simulink model "mcb_stm32_param_est_host_read"  (R2024a)
settings: Solver=FixedStepDiscrete  StartTime=0.0  StopTime=60  RelTol=1e-3
InitFcn:
  | mcb_stm32_param_est_InitFunc(bdroot);
StopFcn:
  | mcb_param_est_StopFunc(bdroot);
values from neighbouring files (symbols this model uses):
  motorParam =     [matlab.mat]
  Speed_per_unit_scaler = motorParam.ratedSpeed    [mcb_stm32_param_est_InitFunc.m]
  Ts = 1/PWM_frequency    (= 5e-05)    [mcb_stm32_param_est_InitFunc.m]    (also in stm32_pmsm_foc_data.m)
undefined symbols (not defined in the file or in its folder): inverter
libraries: instrumentseriallib x5, simulink x5
settings Model: Creator=The MathWorks, Inc.  LastModifiedBy=wsl
settings SolverCC: AlgebraicLoopSolver=TrustRegion  MaxZcPerStep=1
settings DataIOCC: LimitDataPoints=on  SaveFormat=Array  ReturnWorkspaceOutputs=off
settings OptimizationCC: ReuseModelBlockBuffer=off  LifeSpan=1  EfficientTunableParamExpr=on
settings DebuggingCC: UnderspecifiedInitializationDetection=Classic  MergeDetectMultiDrivingBlocksExec=none  SolverPrmCheckMsg=warning  MultiTaskCondExecSysMsg=warning  ParameterOverflowMsg=none  ParameterPrecisionLossMsg=none  UnconnectedInputMsg=warning  UnconnectedOutputMsg=warning  UnconnectedLineMsg=warning  AllowSymbolicDim=off  SubsystemReferenceDiagnosticForUnitTest=warning  SFUnexpectedBacktrackingDiag=warning  SFNoUnconditionalDefaultTransitionDiag=warning  SFExecutionAtInitializationDiag=none  ArithmeticOperatorsInVariantConditions=warning
settings HardwareCC: ProdBitPerPointer=32  ProdLargestAtomicFloat=None  ProdIntDivRoundTo=Undefined  ProdEndianess=Unspecified  ProdWordSize=32  ProdHWDeviceType=32-bit Generic
settings ModelReferenceCC: EnableRefExpFcnMdlSchedulingChecks=on  PropagateSignalLabelsOutOfModel=off
settings SFSimCC: SimUseLocalCustomCode=off  MATLABDynamicMemAlloc=off
settings RTWCC: Description=Real-Time Workshop Embedded Coder  SystemTargetFile=ert.tlc  TemplateMakefile=ert_default_tmf  GenerateReport=on  RTWUseLocalCustomCode=off  IncludeHyperlinkInReport=on  LaunchReport=on  GenerateTraceInfo=on  GenerateTraceReport=on  GenerateTraceReportSl=on  GenerateTraceReportSf=on  GenerateTraceReportEml=on  GPUComputeCapability=3.5  DLArmComputeVersion=19.05
settings CodeAppCC: IgnoreCustomStorageClasses=off  StateflowObjectComments=on  InternalIdentifier=Classic
settings ERTTargetCC: MultiwordLength=2048  GenerateSampleERTMain=on  ERTCustomFileTemplate=example_file_process.tlc  ConvertIfToSwitch=off  SuppressUnreachableDefaultCases=off
settings ConfigComp: CovMetricSettings=dw  CovSaveCumulativeToWorkspaceVar=on  CovSaveSingleToWorkspaceVar=on  CovExternalEMLEnable=off  CovSFcnEnable=off

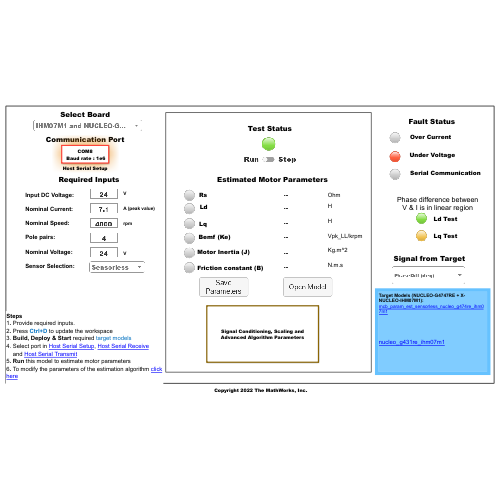
[thumbnail: Simulink's stored preview of the top-level diagram]
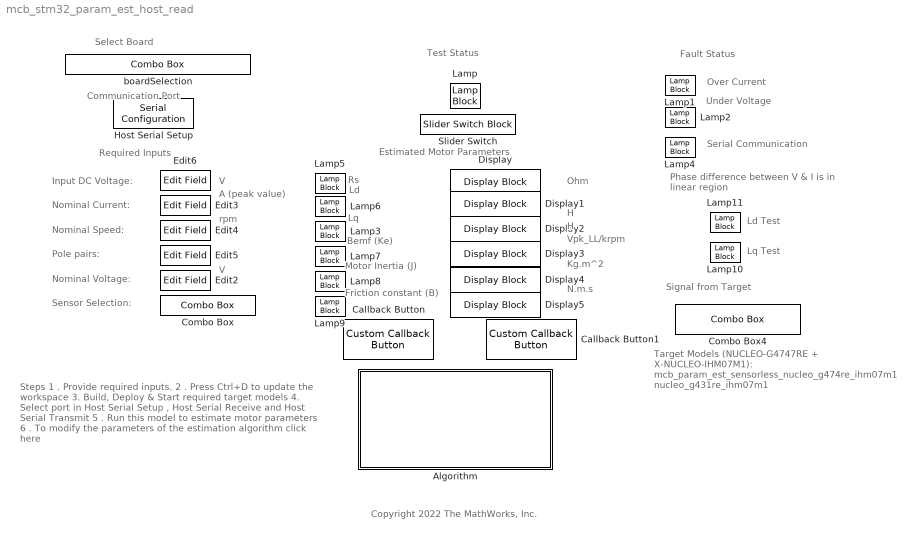
== system mcb_stm32_param_est_host_read ==
  note: Rs
  note: Ld
  note: Lq
  note: Bemf (Ke)
  note: Motor Inertia (J)
  note: Required Inputs
  note: Select Board
  note: Nominal Voltage:
  note: Nominal Current:
  note: Nominal Speed:
  note: rpm
  note: V
  note: A (peak value)
  note: Pole pairs:
  note: Input DC Voltage:
  note: Friction constant (B)
  note: Ohm
  note: H
  note: N.m.s
  note: Over Current
  note: Under Voltage
  note: Serial Communication
  note: Estimated Motor Parameters
  note: Signal from Target
  note: Test Status
  note: Copyright 2022 The MathWorks, Inc.
  note: Communication Port
  note: Sensor Selection:
  note: Steps
      | 1 . Provide required inputs.
      | 2 . Press Ctrl+D to update the workspace
      | 3. Build, Deploy & Start required target models
      | 4. Select port in Host Serial Setup , Host Serial Receive
      | and Host Serial Transmit
      | 5 . Run this model to estimate motor parameters
      | 6 . To modify the parameters of the estimation algorithm click here
  note: Vpk_LL/krpm
  note: H
  note: Kg.m^2
  note: V
  note: Target Models (NUCLEO-G4747RE + X-NUCLEO-IHM07M1):
      | mcb_param_est_sensorless_nucleo_g474re_ihm07m1
      |
      | nucleo_g431re_ihm07m1
  note: Phase difference between
      | V & I is in linear region
  note: Ld Test
  note: Lq Test
  note: Fault Status
  Algorithm : Subsystem
      mask Display: fprintf('Signal Conditioning, Scaling and\nAdvanced Algorithm Parameters')
  Callback Button : CustomCallbackButton  Configuration="{\"components\":[{\"name\":\"BackgroundImageComponent\",\"settings\":{\"image\":{\"size\":[0,0],\"src\":\"default\",\"srcOrientation\":\"Right\"},\"position\":[0,0,1,1]}},{\"name\":\"ButtonStateComponent\",\"settings\":{\"buttonType\":\"momentary\",\"clickFcn\":\"uisave('motorParam');\",\"onValue\":1,\"position\":[0,0,1,1],\"pressDelay\":\"500\",\"pressFcn\":\"\",\"repeatInterval\":\"0\",\"states\":[{\"horizontalAlignment\":\"center\",\"image\":{\"position\":[0,0,1,1],\"src\":\"default\",\"srcOrientation\":\"Right\"},\"label\":{\"color\":[0.01176470588,0.01176470588,0.01176470588,1],\"icon\":{\"size\":[0,0],\"src\":\"default\",\"srcOrientation\":\"Right\"},\"iconPlacement\":\"left\",\"text\":{\"content\":\"Save Parameters\"}},\"labelOffset\":[0,0],\"verticalAlignment\":\"middle\"},{\"horizontalAlignment\":\"center\",\"image\":{\"position\":[0,0,1,1],\"src\":\"default\",\"srcOrientation\":\"Right\"},\"label\":{\"color\":[0.01176470588,0.01176470588,0.01176470588,1],\"icon\":{\"size\":[0,0],\"src\":\"default\",\"srcOrientation\":\"Right\"},\"iconPlacement\":\"left\",\"text\":{\"content\":\"Save Parameters\"}},\"labelOffset\":[0,0],\"verticalAlignment\":\"middle\"},{\"horizontalAlignment\":\"center\",\"image\":{\"position\":[0,0,1,1],\"src\":\"default\",\"srcOrientation\":\"Right\"},\"label\":{\"color\":[0.01176470588,0.01176470588,0.01176470588,1],\"icon\":{\"size\":[0,0],\"src\":\"default\",\"srcOrientation\":\"Right\"},\"iconPlacement\":\"left\",\"text\":{\"content\":\"Save Parameters\"}},\"labelOffset\":[0,0],\"verticalAlignment\":\"middle\"},{\"horizontalAlignment\":\"center\",\"image\":{\"position\":[0,0,1,1],\"src\":\"default\",\"srcOrientation\":\"Right\"},\"label\":{\"color\":[0.01176470588,0.01176470588,0.01176470588,1],\"icon\":{\"size\":[0,0],\"src\":\"default\",\"srcOrientation\":\"Right\"},\"iconPlacement\":\"left\",\"text\":{\"content\":\"Save Parameters\"}},\"labelOffset\":[0,0],\"verticalAlignment\":\"middle\"}]}},{\"name\":\"ForegroundImageComponent\",\"settings\":{\"image\":{\"size\":[0,0],\"src\":\"default\",\"srcOrientation\":\"Right\"},\"isForeground\":1,\"position\":[0,0,1,1]}}],\"settings\":{\"BindingType\":\"standalone\",\"backgroundColor\":[244,244,244,1],\"backgroundOffset\":0.2,\"backgroundOpacity\":1,\"fixedAspectRatio\":\"off\",\"foregroundColor\":[0.01176470588,0.01176470588,0.01176470588,1],\"migratedFromLegacy\":true,\"useBackgroundColor\":true,\"variant\":\"callback\",\"version\":\"R2023a\"},\"type\":\"Button\"}"  CustomBackgroundColor="{\"color\":[0.9568627451,0.9568627451,0.9568627451],\"show\":true}"
  Callback Button1 : CustomCallbackButton  Configuration="{\"components\":[{\"name\":\"BackgroundImageComponent\",\"settings\":{\"image\":{\"size\":[0,0],\"src\":\"default\",\"srcOrientation\":\"Right\"},\"position\":[0,0,1,1]}},{\"name\":\"ButtonStateComponent\",\"settings\":{\"buttonType\":\"momentary\",\"clickFcn\":\"hdl = new_system;\\nopen_system(hdl);\\nblkHdl = add_block('mcblib\\/Electrical Systems\\/Motors\\/Interior PMSM', [get_param(hdl,'Name'),'\\/Interior PMSM']);\\nopen_system(hdl);\\nset_param(blkHdl,'P','motorParam.p');\\nset_param(blkHdl,'Rs','motorParam.Rs');\\nset_param(blkHdl,'Ldq','[motorParam.Ld motorParam.Lq]');\\nset_param(blkHdl,'KConstText','Back-emf constant (Ke):');\\nset_param(blkHdl,'Ke','motorParam.Ke');\\nset_param(blkHdl,'mechanical','[motorParam.J, motorParam.B, 0]');\",\"onValue\":1,\"position\":[0,0,1,1],\"pressDelay\":\"500\",\"pressFcn\":\"\",\"repeatInterval\":\"0\",\"states\":[{\"horizontalAlignment\":\"center\",\"image\":{\"position\":[0,0,1,1],\"src\":\"default\",\"srcOrientation\":\"Right\"},\"label\":{\"color\":[0.01176470588,0.01176470588,0.01176470588,1],\"icon\":{\"size\":[0,0],\"src\":\"default\",\"srcOrientation\":\"Right\"},\"iconPlacement\":\"left\",\"text\":{\"content\":\"Open Model\"}},\"labelOffset\":[0,0],\"verticalAlignment\":\"middle\"},{\"horizontalAlignment\":\"center\",\"image\":{\"position\":[0,0,1,1],\"src\":\"default\",\"srcOrientation\":\"Right\"},\"label\":{\"color\":[0.01176470588,0.01176470588,0.01176470588,1],\"icon\":{\"size\":[0,0],\"src\":\"default\",\"srcOrientation\":\"Right\"},\"iconPlacement\":\"left\",\"text\":{\"content\":\"Open Model\"}},\"labelOffset\":[0,0],\"verticalAlignment\":\"middle\"},{\"horizontalAlignment\":\"center\",\"image\":{\"position\":[0,0,1,1],\"src\":\"default\",\"srcOrientation\":\"Right\"},\"label\":{\"color\":[0.01176470588,0.01176470588,0.01176470588,1],\"icon\":{\"size\":[0,0],\"src\":\"default\",\"srcOrientation\":\"Right\"},\"iconPlacement\":\"left\",\"text\":{\"content\":\"Open Model\"}},\"labelOffset\":[0,0],\"verticalAlignment\":\"middle\"},{\"horizontalAlignment\":\"center\",\"image\":{\"position\":[0,0,1,1],\"src\":\"default\",\"srcOrientation\":\"Right\"},\"label\":{\"color\":[0.01176470588,0.01176470588,0.01176470588,1],\"icon\":{\"size\":[0,0],\"src\":\"default\",\"srcOrientation\":\"Right\"},\"iconPlacement\":\"left\",\"text\":{\"content\":\"Open Model\"}},\"labelOffset\":[0,0],\"verticalAlignment\":\"middle\"}]}},{\"name\":\"ForegroundImageComponent\",\"settings\":{\"image\":{\"size\":[0,0],\"src\":\"default\",\"srcOrientation\":\"Right\"},\"isForeground\":1,\"position\":[0,0,1,1]}}],\"settings\":{\"BindingType\":\"standalone\",\"backgroundColor\":[244,244,244,1],\"backgroundOffset\":0.2,\"backgroundOpacity\":1,\"fixedAspectRatio\":\"off\",\"foregroundColor\":[0.01176470588,0.01176470588,0.01176470588,1],\"migratedFromLegacy\":true,\"useBackgroundColor\":true,\"variant\":\"callback\",\"version\":\"R2023a\"},\"type\":\"Button\"}"  CustomBackgroundColor="{\"color\":[0.9568627451,0.9568627451,0.9568627451],\"show\":true}"
  Combo Box : ComboBox  LabelPosition=Hide  SelectedLabel=Sensorless
      settings: Values={{'Sensorless'}, 2}
  Combo Box4 : ComboBox  LabelPosition=Hide  SelectedLabel=PhaseDiff (deg)
      settings: Values={{'Vd', 'Id', 'Vq', 'Iq', 'Ia', 'Ib', 'Theta', 'Speed', 'Vq_Meas', 'Vd_Meas', 'Vdc_Meas', 'PhaseDiff (deg)'}, [1 8 0 7 9 10 6 5 3 4 2 11]}
  Display{,1..5} (6 alike) : DisplayBlock  LabelPosition=Hide  Transparency=1  Opacity=0.001
  Edit{2..6} (5 alike) : EditField  LabelPosition=Hide  ShowInitialText=on  Alignment=Center
  Host Serial Setup : instrumentseriallib/Serial Configuration  Priority=-99  PortSel=COM8  Port=COM8  ComPort=COM8  BaudRate=1e6  DataBits=8  Parity=none  StopBits=1  ByteOrder=little-endian  FlowControl=none  Timeout=1  SimulateUsing=Interpreted execution  BlockInModel=on  aMode=5
  Lamp{,1..11} (12 alike) : LampBlock  LabelPosition=Hide
  Slider Switch : SliderSwitchBlock  LabelPosition=Hide
      settings: Values={{'Run', 'Stop'}, [1 0]}
  boardSelection : ComboBox  LabelPosition=Hide  SelectedLabel=IHM07M1 and NUCLEO-G474RE
      settings: Values={{'IHM07M1 and NUCLEO-G474RE'}, 2}

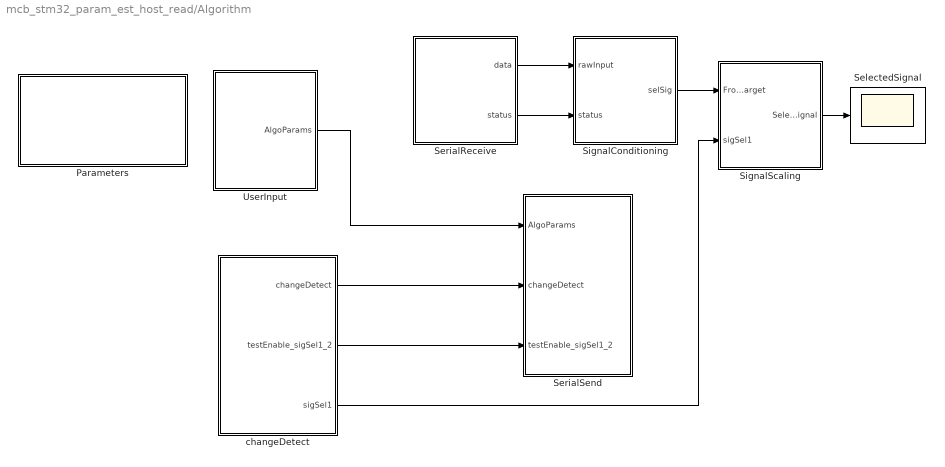
== system mcb_stm32_param_est_host_read/Algorithm ==
  Parameters : Subsystem
      mask Display: fprintf('Advanced Algorithm Parameters')
  SelectedSignal : Scope
  SerialReceive : Subsystem  Variant=on  VariantControlMode=label  LabelModeActiveChoice=Floating_Point_Target
  SerialSend : Subsystem  VariantControl=Choice
  SignalConditioning : Subsystem
  SignalScaling : Subsystem
  UserInput : Subsystem
  changeDetect : Subsystem
  wires:
  changeDetect/1(changeDetect) -> SerialSend/2(changeDetect)
  changeDetect/2("testEnable_sigSel1_2 ") -> SerialSend/3(testEnable_sigSel1_2)
  changeDetect/3(sigSel1) -> SignalScaling/2(sigSel1)
  SignalConditioning/1(selSig) -> SignalScaling/1(FromTarget)
  UserInput/1(AlgoParams) -> SerialSend/1(AlgoParams)
  SerialReceive/1(data) -> SignalConditioning/1(rawInput)
  SerialReceive/2(status) -> SignalConditioning/2(status)
  SignalScaling/1(SelectedSignal) -> SelectedSignal/1

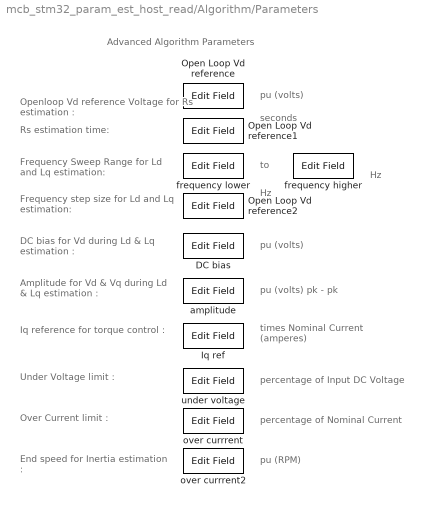
== system mcb_stm32_param_est_host_read/Algorithm/Parameters ==
  note: Openloop Vd reference Voltage
      | for Rs estimation :
  note: pu (volts)
  note: Frequency Sweep Range for Ld and Lq estimation:
  note: to
  note: Hz
  note: DC bias for Vd during Ld & Lq estimation :
  note: Amplitude for Vd & Vq during Ld & Lq estimation :
  note: Iq reference for torque control :
  note: times Nominal Current (amperes)
  note: Under Voltage limit :
  note: percentage of Input DC Voltage
  note: Over Current limit :
  note: percentage of Nominal Current
  note: Rs estimation time:
  note: seconds
  note: Advanced Algorithm Parameters
  note: Frequency step size for Ld and Lq estimation:
  note: Hz
  note: End speed for Inertia estimation :
  note: pu (RPM)
  note: pu (volts)
  note: pu (volts) pk - pk
  DC bias : EditField  LabelPosition=Hide  ShowInitialText=on  Alignment=Center
  Iq ref : EditField  LabelPosition=Hide  ShowInitialText=on  Alignment=Center
  Open Loop Vd reference : EditField  LabelPosition=Hide  ShowInitialText=on  Alignment=Center
  Open Loop Vd reference1 : EditField  LabelPosition=Hide  ShowInitialText=on  Alignment=Center
  Open Loop Vd reference2 : EditField  LabelPosition=Hide  ShowInitialText=on  Alignment=Center
  amplitude : EditField  LabelPosition=Hide  ShowInitialText=on  Alignment=Center
  frequency higher : EditField  LabelPosition=Hide  ShowInitialText=on  Alignment=Center
  frequency lower : EditField  LabelPosition=Hide  ShowInitialText=on  Alignment=Center
  over currrent : EditField  LabelPosition=Hide  ShowInitialText=on  Alignment=Center
  over currrent2 : EditField  LabelPosition=Hide  ShowInitialText=on  Alignment=Center
  under voltage : EditField  LabelPosition=Hide  ShowInitialText=on  Alignment=Center

== system mcb_stm32_param_est_host_read/Algorithm/SerialReceive ==
  Fixed_Point_Target : Subsystem  VariantControl=Fixed_Point_Target
  Floating_Point_Target : Subsystem  VariantControl=Floating_Point_Target
  data : Outport
  status : Outport  Port=2

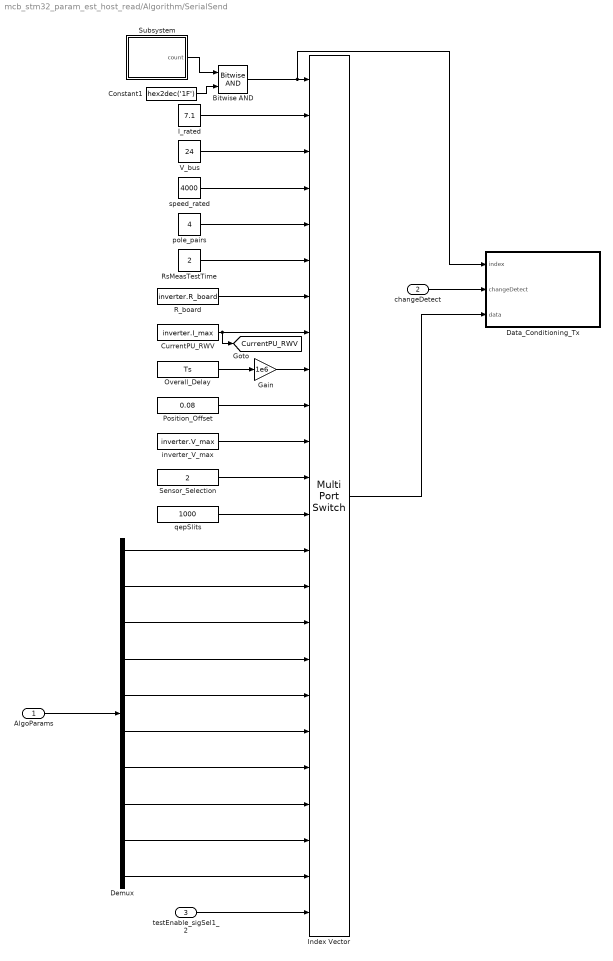
== system mcb_stm32_param_est_host_read/Algorithm/SerialSend ==
  AlgoParams : Inport
  changeDetect : Inport  Port=2
  testEnable_sigSel1_2 : Inport  Port=3
  Bitwise AND : simulink/Logic and Bit Operations/Bitwise Operator  logicop=AND  UseBitMask=off  NumInputPorts=2  BitMask=bin2dec('00001111')  BitMaskRealWorld=Stored Integer
  Constant1 : Constant  Value=hex2dec('1F')  OutDataTypeStr=uint8  SampleTime=-1
  CurrentPU_RWV : Constant  Value=inverter.I_max  OutDataTypeStr=single  SampleTime=-1
  Data_Conditioning_Tx : Subsystem  Variant=on  VariantControlMode=label  LabelModeActiveChoice=Floating_Point_Target
  Demux : Demux  Outputs=10
  Gain : Gain  Gain=1e6  OutDataTypeStr=single  RndMeth=Simplest
  I_rated : Constant  Value=7.1  OutMin=[0]  OutMax=[25000]  OutDataTypeStr=single  SampleTime=-1
  Index Vector : MultiPortSwitch  Inputs=23  OutDataTypeStr=single  RndMeth=Simplest  SaturateOnIntegerOverflow=off  InputSameDT=off
  Overall_Delay : Constant  Value=Ts  OutDataTypeStr=single  SampleTime=-1
  Position_Offset : Constant  Value=0.08  OutMin=[0]  OutMax=[1]  OutDataTypeStr=single  SampleTime=-1
  R_board : Constant  Value=inverter.R_board  OutDataTypeStr=single  SampleTime=-1
  RsMeasTestTime : Constant  Value=2  OutMin=[0.2]  OutMax=[25000]  OutDataTypeStr=single  SampleTime=-1
  Sensor_Selection : Constant  Value=2  OutDataTypeStr=single  SampleTime=-1
  Subsystem : Subsystem  mask(Counter){upperLimit=23, sampleTime=1e-3}
      mask prompts: upperLimit "Upper Limit"; sampleTime "Sample Time"
      mask help: Conter starts from 1 and reaches Upper Limit using given sample time in steps of 1.
  V_bus : Constant  Value=24  OutMin=[0]  OutMax=[25000]  OutDataTypeStr=single  SampleTime=-1
  inverter_V_max : Constant  Value=inverter.V_max  OutDataTypeStr=single  SampleTime=-1
  pole_pairs : Constant  Value=4  OutMin=[1]  OutMax=[25000]  OutDataTypeStr=single  SampleTime=-1
  qepSlits : Constant  Value=1000  OutDataTypeStr=single  SampleTime=-1
  speed_rated : Constant  Value=4000  OutMin=[0]  OutMax=[25000]  OutDataTypeStr=single  SampleTime=-1
  tag scope: CurrentPU_RWV=global
  wires:
  pole_pairs/1 -> Index Vector/5
  V_bus/1 -> Index Vector/3
  speed_rated/1 -> Index Vector/4
  Constant1/1 -> Bitwise AND/2
  RsMeasTestTime/1 -> Index Vector/6
  Bitwise AND/1 -> Data_Conditioning_Tx/1(index), Index Vector/1
  R_board/1 -> Index Vector/7
  CurrentPU_RWV/1 -> [CurrentPU_RWV], Index Vector/8
  Overall_Delay/1 -> Gain/1
  Gain/1 -> Index Vector/9
  I_rated/1 -> Index Vector/2
  inverter_V_max/1 -> Index Vector/11
  Sensor_Selection/1 -> Index Vector/12
  Position_Offset/1 -> Index Vector/10
  qepSlits/1 -> Index Vector/13
  changeDetect/1 -> Data_Conditioning_Tx/2(changeDetect)
  Index Vector/1 -> Data_Conditioning_Tx/3(data)
  AlgoParams/1 -> Demux/1
  Subsystem/1(count) -> Bitwise AND/1
  Demux/1 -> Index Vector/14
  Demux/2 -> Index Vector/15
  Demux/3 -> Index Vector/16
  Demux/4 -> Index Vector/17
  Demux/5 -> Index Vector/18
  Demux/6 -> Index Vector/19
  Demux/7 -> Index Vector/20
  Demux/8 -> Index Vector/21
  Demux/9 -> Index Vector/22
  Demux/10 -> Index Vector/23
  testEnable_sigSel1_2/1 -> Index Vector/24

== system mcb_stm32_param_est_host_read/Algorithm/SignalConditioning ==
  rawInput : Inport
  status : Inport  Port=2
  Data_Conditioning1 : MATLAB Function  TreatAsAtomicUnit=on
  Data_Conditioning2 : MATLAB Function  TreatAsAtomicUnit=on
  ErrorConditions : MATLAB Function  TreatAsAtomicUnit=on
  LatchIdx : Subsystem
  Subsystem1 : Subsystem
  selSig : Outport
  wires:
  Subsystem1/1(errorID) -> ErrorConditions/3(errorID)
  Data_Conditioning1/2(estParam) -> Subsystem1/2(estimatedParameter)
  Data_Conditioning1/1(estParamIdx) -> LatchIdx/2(estParIdx), ErrorConditions/2(idx), Subsystem1/1(Idx)
  rawInput/1 -> Data_Conditioning2/1(rawInput), Data_Conditioning1/2(rawInput)
  Data_Conditioning2/1(selSignal) -> selSig/1
  status/1 -> ErrorConditions/1(status), LatchIdx/1(status), Data_Conditioning1/1(unused)

== system mcb_stm32_param_est_host_read/Algorithm/SignalScaling ==
  FromTarget : Inport
  sigSel1 : Inport  Port=2
  Data Type Conversion : DataTypeConversion  OutDataTypeStr=single  RndMeth=Simplest  SaturateOnIntegerOverflow=off
  PU2RWV : Subsystem
  To Workspace3 : ToWorkspace  VariableName=SignalsScaled  SaveFormat=Timeseries  SampleTime=-1
  SelectedSignal : Outport
  wires:
  FromTarget/1 -> Data Type Conversion/1  "FreqTrgt/Speed"
  sigSel1/1 -> PU2RWV/2(SelTestHost)
  PU2RWV/1(RWV) -> SelectedSignal/1, To Workspace3/1  "SelectedSignal"
  Data Type Conversion/1 -> PU2RWV/1(SigFromTarget)

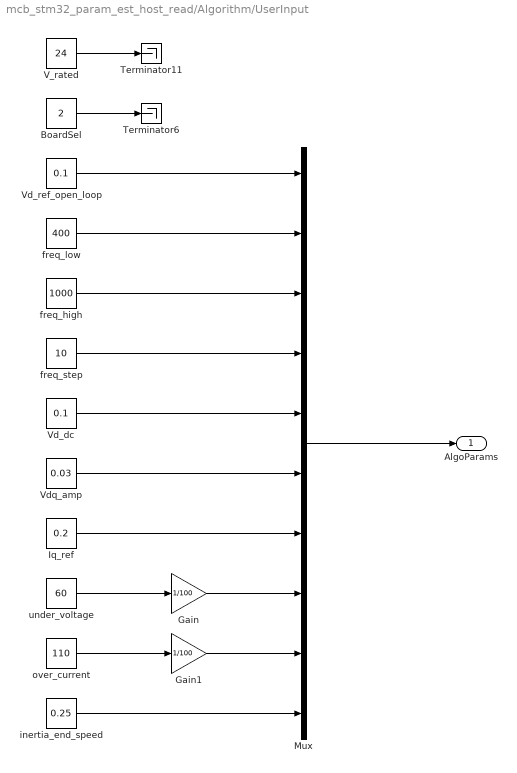
== system mcb_stm32_param_est_host_read/Algorithm/UserInput ==
  BoardSel : Constant  Value=2  OutDataTypeStr=single  SampleTime=-1
  Gain : Gain  Gain=1/100  OutDataTypeStr=single  RndMeth=Simplest
  Gain1 : Gain  Gain=1/100  OutDataTypeStr=single  RndMeth=Simplest
  Iq_ref : Constant  Value=0.2  OutMin=[0.05]  OutMax=[0.5]  OutDataTypeStr=single  SampleTime=-1
  Mux : Mux  Inputs=10
  Terminator11 : Terminator
  Terminator6 : Terminator
  V_rated : Constant  Value=24  OutMin=[0]  OutMax=[100000]  OutDataTypeStr=single  SampleTime=-1
  Vd_dc : Constant  Value=0.1  OutMin=[0.01]  OutMax=[0.5]  OutDataTypeStr=single  SampleTime=-1
  Vd_ref_open_loop : Constant  Value=0.1  OutMin=[0.01]  OutMax=[0.5]  OutDataTypeStr=single  SampleTime=-1
  Vdq_amp : Constant  Value=0.03  OutMin=[1e-3]  OutMax=[0.9]  OutDataTypeStr=single  SampleTime=-1
  freq_high : Constant  Value=1000  OutMin=[100]  OutMax=[10000]  OutDataTypeStr=single  SampleTime=-1
  freq_low : Constant  Value=400  OutMin=[100]  OutMax=[10000]  OutDataTypeStr=single  SampleTime=-1
  freq_step : Constant  Value=10  OutMin=[10]  OutMax=[10000]  OutDataTypeStr=single  SampleTime=-1
  inertia_end_speed : Constant  Value=0.25  OutMin=[0.25]  OutMax=[0.7]  OutDataTypeStr=single  SampleTime=-1
  over_current : Constant  Value=110  OutMin=[20]  OutMax=[150]  OutDataTypeStr=single  SampleTime=-1
  under_voltage : Constant  Value=60  OutMin=[10]  OutMax=[100]  OutDataTypeStr=single  SampleTime=-1
  AlgoParams : Outport
  wires:
  BoardSel/1 -> Terminator6/1
  V_rated/1 -> Terminator11/1
  under_voltage/1 -> Gain/1
  over_current/1 -> Gain1/1
  Mux/1 -> AlgoParams/1
  Gain/1 -> Mux/8
  Gain1/1 -> Mux/9
  freq_high/1 -> Mux/3
  freq_low/1 -> Mux/2
  freq_step/1 -> Mux/4
  Vd_ref_open_loop/1 -> Mux/1
  Vd_dc/1 -> Mux/5
  Vdq_amp/1 -> Mux/6
  Iq_ref/1 -> Mux/7
  inertia_end_speed/1 -> Mux/10

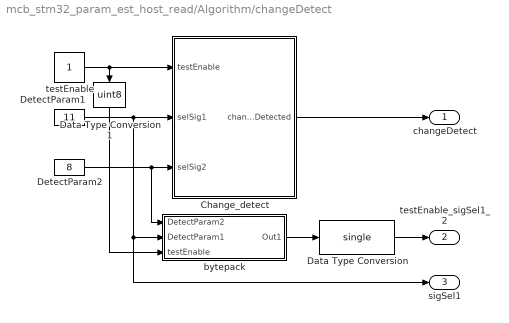
== system mcb_stm32_param_est_host_read/Algorithm/changeDetect ==
  Change_detect : Subsystem
  Data Type Conversion : DataTypeConversion  OutDataTypeStr=single  SaturateOnIntegerOverflow=off  RndMeth=Floor
  Data Type Conversion1 : DataTypeConversion  OutDataTypeStr=uint8  SaturateOnIntegerOverflow=off  RndMeth=Floor
  DetectParam1 : Constant  Value=11  OutDataTypeStr=uint8  SampleTime=-1
  DetectParam2 : Constant  Value=8  OutDataTypeStr=uint8  SampleTime=-1
  bytepack : Subsystem
  testEnable : Constant  OutDataTypeStr=boolean  SampleTime=-1
  changeDetect : Outport
  "testEnable_sigSel1_2 " : Outport  Port=2
  sigSel1 : Outport  Port=3
  wires:
  DetectParam1/1 -> sigSel1/1, bytepack/2(DetectParam1), Change_detect/2(selSig1)
  Change_detect/1(changeDetected) -> changeDetect/1
  testEnable/1 -> Data Type Conversion1/1, Change_detect/1(testEnable)
  bytepack/1(Out1) -> Data Type Conversion/1
  Data Type Conversion/1 -> "testEnable_sigSel1_2 "/1
  Data Type Conversion1/1 -> bytepack/3(testEnable)
  DetectParam2/1 -> bytepack/1(DetectParam2), Change_detect/3(selSig2)

== system mcb_stm32_param_est_host_read/Algorithm/SerialReceive/Fixed_Point_Target ==
  Constant : Constant  Value=404  OutDataTypeStr=Inherit: Inherit via back propagation
  Data Type Conversion1 : DataTypeConversion  OutDataTypeStr=single  RndMeth=Simplest  SaturateOnIntegerOverflow=off
  Data Type Conversion6 : DataTypeConversion  OutDataTypeStr=fixdt(1,32,25)  ConvertRealWorld=Stored Integer (SI)  RndMeth=Simplest  SaturateOnIntegerOverflow=off
  Host Serial Receive : instrumentseriallib/Serial Receive  PortSel=COM8  Port=COM8  ComPort=COM8  DataType=single  SaveDataType=uint8  ToggleHeader=on  Header='SSSS'  ToggleDataSize=on  DataSize=[600 2]  ToggleTerminator=on  Terminator=Custom terminator  CustomTerminator='EEEE'  InputFormat=Row major  EnableBlockingMode=on  ActionDataUnavailable=Output custom value  ActionWhenDataUnavailable=Output custom value  CustomValue=404  SampleTime=600*Ts  SimulateUsing=Interpreted execution  BlockInModel=on  aMode=5
  LatchZero : Subsystem
  checkStatus : MATLAB Function  TreatAsAtomicUnit=on
  data : Outport  VectorParamsAs1DForOutWhenUnconnected=off
  status : Outport  Port=2  VectorParamsAs1DForOutWhenUnconnected=off
  wires:
  LatchZero/1(status) -> status/1
  Data Type Conversion1/1 -> data/1
  Data Type Conversion6/1 -> Data Type Conversion1/1
  Host Serial Receive/1 -> Data Type Conversion6/1, checkStatus/1(Data)
  checkStatus/1(Status) -> LatchZero/1(Status)
  Constant/1 -> checkStatus/2(ErrorCode)

== system mcb_stm32_param_est_host_read/Algorithm/SerialReceive/Floating_Point_Target ==
  Constant : Constant  Value=single(404)
  Host Serial Receive : instrumentseriallib/Serial Receive  PortSel=COM8  Port=COM8  ComPort=COM8  DataType=single  SaveDataType=uint8  ToggleHeader=on  Header='SSSS'  ToggleDataSize=on  DataSize=[600 2]  ToggleTerminator=on  Terminator=Custom terminator  CustomTerminator='EEEE'  InputFormat=Row major  EnableBlockingMode=on  ActionDataUnavailable=Output last received value  ActionWhenDataUnavailable=Output last received value  CustomValue=404  SampleTime=600*Ts  SimulateUsing=Interpreted execution  BlockInModel=on  aMode=5
  LatchZero : Subsystem
  checkStatus : MATLAB Function  TreatAsAtomicUnit=on
  data : Outport  VectorParamsAs1DForOutWhenUnconnected=off
  status : Outport  Port=2  VectorParamsAs1DForOutWhenUnconnected=off
  wires:
  checkStatus/1(Status) -> LatchZero/1(Status)
  Host Serial Receive/1 -> checkStatus/1(Data), data/1
  LatchZero/1(status) -> status/1
  Constant/1 -> checkStatus/2(ErrorCode)

== system mcb_stm32_param_est_host_read/Algorithm/SerialSend/Data_Conditioning_Tx ==
  index : Inport
  changeDetect : Inport  Port=2
  data : Inport  Port=3
  Fixed_Point_Target : Subsystem  VariantControl=Fixed_Point_Target
  Floating_Point_Target : Subsystem  VariantControl=Floating_Point_Target

== system mcb_stm32_param_est_host_read/Algorithm/SerialSend/Subsystem ==
  Constant : Constant  OutDataTypeStr=uint8  SampleTime=sampleTime
  Constant1 : Constant  Value=0  OutDataTypeStr=uint8  SampleTime=sampleTime
  Sum : Sum  Inputs=++|  OutDataTypeStr=uint8  AccumDataTypeStr=uint8  RndMeth=Simplest
  Switch : Switch  Criteria=u2 > Threshold  Threshold=upperLimit-1  OutDataTypeStr=uint8  RndMeth=Simplest  SaturateOnIntegerOverflow=off  InputSameDT=off
  Unit Delay : UnitDelay  SampleTime=-1  HasFrameUpgradeWarning=on
  count : Outport
  wires:
  Constant1/1 -> Switch/1
  Sum/1 -> count/1, Unit Delay/1
  Unit Delay/1 -> Switch/2, Sum/1
  Switch/1 -> Sum/2
  Constant/1 -> Switch/3

== system mcb_stm32_param_est_host_read/Algorithm/SignalConditioning/LatchIdx ==
  note: Note: This subsystem is used to glow status LEDs for each parameter test
  status : Inport
  estParIdx : Inport  Port=2
  AND : Logic  AllPortsSameDT=off  OutDataTypeStr=boolean
  Compare To Constant : simulink/Logic and Bit Operations/Compare To Constant  relop=~=  const=9  OutDataTypeStr=boolean
  Enabled Subsystem : Subsystem  TreatAsAtomicUnit=on
  Terminator : Terminator
  wires:
  estParIdx/1 -> Enabled Subsystem/1(status), Compare To Constant/1
  AND/1 -> Enabled Subsystem/Enable
  Compare To Constant/1 -> AND/1
  Enabled Subsystem/1(Idx) -> Terminator/1
  status/1 -> AND/2

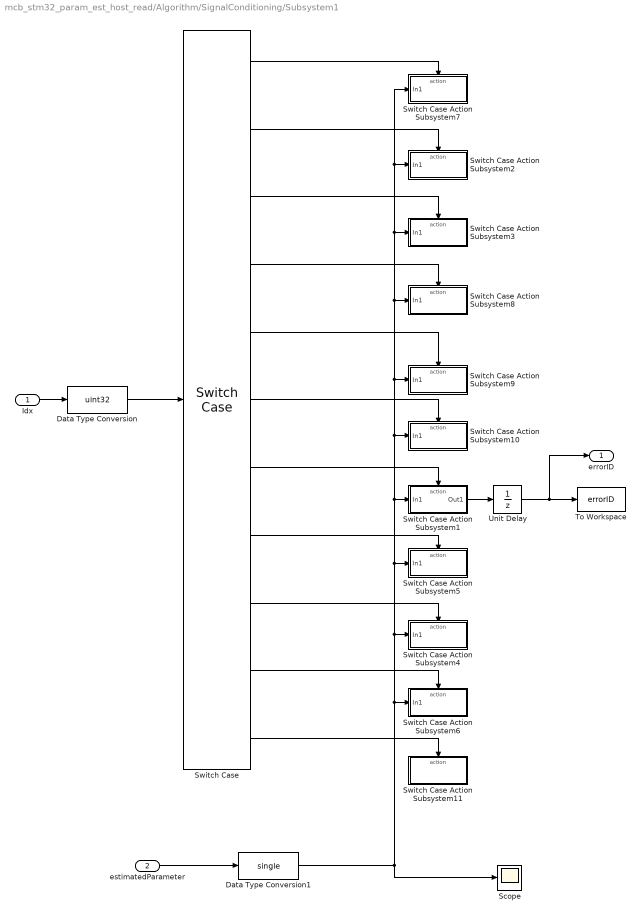
== system mcb_stm32_param_est_host_read/Algorithm/SignalConditioning/Subsystem1 ==
  Idx : Inport
  estimatedParameter : Inport  Port=2
  Data Type Conversion : DataTypeConversion  OutDataTypeStr=uint32  RndMeth=Nearest  SaturateOnIntegerOverflow=off
  Data Type Conversion1 : DataTypeConversion  OutDataTypeStr=single  RndMeth=Simplest  SaturateOnIntegerOverflow=off
  Scope : Scope
  Switch Case : SwitchCase  CaseConditions={2 3 4 5 6 7 8 0 1 9}
  Switch Case Action Subsystem1 : Subsystem  TreatAsAtomicUnit=on
  Switch Case Action Subsystem10 : Subsystem  TreatAsAtomicUnit=on
  Switch Case Action Subsystem11 : Subsystem  TreatAsAtomicUnit=on
  Switch Case Action Subsystem2 : Subsystem  TreatAsAtomicUnit=on
  Switch Case Action Subsystem3 : Subsystem  TreatAsAtomicUnit=on
  Switch Case Action Subsystem4 : Subsystem  TreatAsAtomicUnit=on
  Switch Case Action Subsystem5 : Subsystem  TreatAsAtomicUnit=on
  Switch Case Action Subsystem6 : Subsystem  TreatAsAtomicUnit=on
  Switch Case Action Subsystem7 : Subsystem  TreatAsAtomicUnit=on
  Switch Case Action Subsystem8 : Subsystem  TreatAsAtomicUnit=on
  Switch Case Action Subsystem9 : Subsystem  TreatAsAtomicUnit=on
  To Workspace : ToWorkspace  VariableName=errorID  SampleTime=-1
      settings: MaxDataPoints=1  Save2DSignal=2-D array (concatenate along first dimension)
  Unit Delay : UnitDelay  SampleTime=-1  HasFrameUpgradeWarning=on
  errorID : Outport
  wires:
  Switch Case/7 -> Switch Case Action Subsystem1/Action
  Switch Case/8 -> Switch Case Action Subsystem5/Action
  Switch Case Action Subsystem1/1(Out1) -> Unit Delay/1
  Switch Case/1 -> Switch Case Action Subsystem7/Action
  Data Type Conversion/1 -> Switch Case/1
  Idx/1 -> Data Type Conversion/1
  Switch Case/3 -> Switch Case Action Subsystem3/Action
  Switch Case/4 -> Switch Case Action Subsystem8/Action
  Switch Case/2 -> Switch Case Action Subsystem2/Action
  Switch Case/5 -> Switch Case Action Subsystem9/Action
  Switch Case/6 -> Switch Case Action Subsystem10/Action
  Unit Delay/1 -> errorID/1, To Workspace/1
  estimatedParameter/1 -> Data Type Conversion1/1
  Data Type Conversion1/1 -> Switch Case Action Subsystem7/1(In1), Switch Case Action Subsystem2/1(In1), Switch Case Action Subsystem3/1(In1), Switch Case Action Subsystem8/1(In1), Switch Case Action Subsystem9/1(In1), Switch Case Action Subsystem10/1(In1), Switch Case Action Subsystem1/1(In1), Switch Case Action Subsystem5/1(In1), Switch Case Action Subsystem4/1(In1), Switch Case Action Subsystem6/1(In1), Scope/1
  Switch Case/9 -> Switch Case Action Subsystem4/Action
  Switch Case/10 -> Switch Case Action Subsystem6/Action
  Switch Case/11 -> Switch Case Action Subsystem11/Action

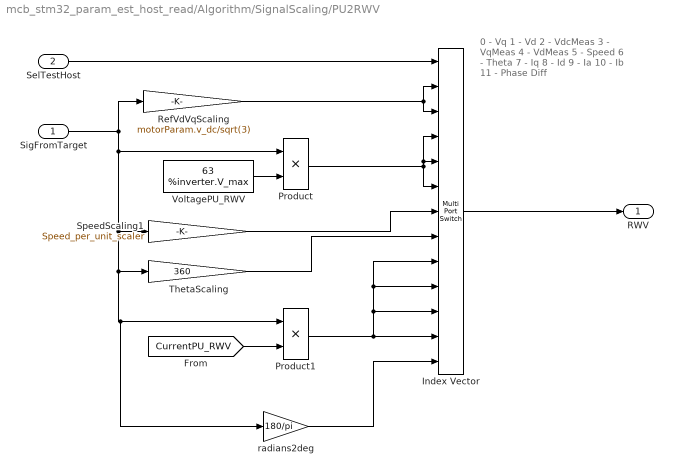
== system mcb_stm32_param_est_host_read/Algorithm/SignalScaling/PU2RWV ==
  note: 0 - Vq
      |
      | 1 - Vd
      | 2 - VdcMeas
      |
      | 3 - VqMeas
      |
      | 4 - VdMeas
      |
      | 5 - Speed
      | 6 - Theta
      |
      | 7 - Iq
      | 8 - Id
      | 9 - Ia
      | 10 - Ib
      | 11 - Phase Diff
  SigFromTarget : Inport
  SelTestHost : Inport  Port=2
  Index Vector : MultiPortSwitch  DataPortOrder=Zero-based contiguous  Inputs=12  DiagnosticForDefault=Warning  zeroidx=on  SaturateOnIntegerOverflow=off  InputSameDT=off
  Product : Product
  Product1 : Product
  RefVdVqScaling : Gain  Gain=motorParam.v_dc/sqrt(3)
  SpeedScaling1 : Gain  Gain=Speed_per_unit_scaler
  ThetaScaling : Gain  Gain=360
  VoltagePU_RWV : Constant  Value=63 %inverter.V_max  OutDataTypeStr=single  SampleTime=-1
  radians2deg : Gain  Gain=180/pi
  RWV : Outport  VectorParamsAs1DForOutWhenUnconnected=off
  wires:
  Index Vector/1 -> RWV/1
  SelTestHost/1 -> Index Vector/1
  RefVdVqScaling/1 -> Index Vector/3, Index Vector/2
  Product1/1 -> Index Vector/11, Index Vector/10, Index Vector/9, Index Vector/12
  Product/1 -> Index Vector/4, Index Vector/5, Index Vector/6
  ThetaScaling/1 -> Index Vector/8
  SpeedScaling1/1 -> Index Vector/7
  SigFromTarget/1 -> radians2deg/1, Product1/1, ThetaScaling/1, SpeedScaling1/1, Product/1, RefVdVqScaling/1
  VoltagePU_RWV/1 -> Product/2
  [CurrentPU_RWV] -> Product1/2
  radians2deg/1 -> Index Vector/13

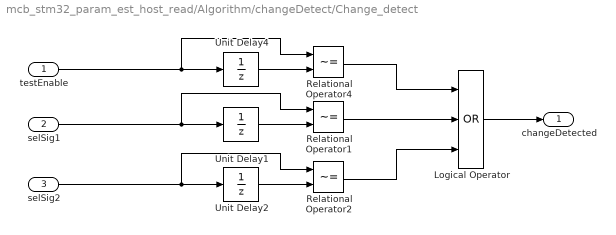
== system mcb_stm32_param_est_host_read/Algorithm/changeDetect/Change_detect ==
  testEnable : Inport
  selSig1 : Inport  Port=2
  selSig2 : Inport  Port=3
  Logical Operator : Logic  Operator=OR  Inputs=3  AllPortsSameDT=off  OutDataTypeStr=boolean
  Relational Operator1 : RelationalOperator  Operator=~=  OutDataTypeStr=boolean  InputSameDT=off
  Relational Operator2 : RelationalOperator  Operator=~=  OutDataTypeStr=boolean  InputSameDT=off
  Relational Operator4 : RelationalOperator  Operator=~=  OutDataTypeStr=boolean  InputSameDT=off
  Unit Delay1 : UnitDelay  InitialCondition=3  SampleTime=-1  HasFrameUpgradeWarning=on
  Unit Delay2 : UnitDelay  InitialCondition=2  SampleTime=-1  HasFrameUpgradeWarning=on
  Unit Delay4 : UnitDelay  SampleTime=-1  HasFrameUpgradeWarning=on
  changeDetected : Outport  VectorParamsAs1DForOutWhenUnconnected=off
  wires:
  selSig1/1 -> Relational Operator1/1, Unit Delay1/1
  Relational Operator1/1 -> Logical Operator/2
  Unit Delay1/1 -> Relational Operator1/2
  Logical Operator/1 -> changeDetected/1
  Unit Delay2/1 -> Relational Operator2/2
  Relational Operator2/1 -> Logical Operator/3
  selSig2/1 -> Unit Delay2/1, Relational Operator2/1
  Unit Delay4/1 -> Relational Operator4/2
  Relational Operator4/1 -> Logical Operator/1
  testEnable/1 -> Unit Delay4/1, Relational Operator4/1

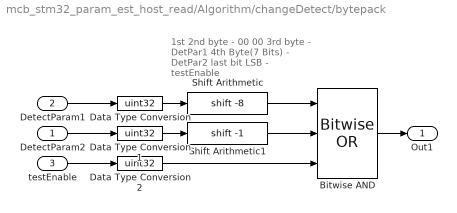
== system mcb_stm32_param_est_host_read/Algorithm/changeDetect/bytepack ==
  note: 1st 2nd byte - 00 00
      | 3rd byte - DetPar1
      | 4th Byte(7 Bits) - DetPar2
      | last bit LSB - testEnable
  DetectParam2 : Inport
  DetectParam1 : Inport  Port=2
  testEnable : Inport  Port=3
  Bitwise AND : simulink/Logic and Bit Operations/Bitwise Operator  logicop=OR  UseBitMask=off  NumInputPorts=3  BitMask=bin2dec('00001111')  BitMaskRealWorld=Stored Integer
  Data Type Conversion : DataTypeConversion  OutDataTypeStr=uint32  RndMeth=Simplest  SaturateOnIntegerOverflow=off
  Data Type Conversion1 : DataTypeConversion  OutDataTypeStr=uint32  RndMeth=Simplest  SaturateOnIntegerOverflow=off
  Data Type Conversion2 : DataTypeConversion  OutDataTypeStr=uint32  RndMeth=Simplest  SaturateOnIntegerOverflow=off
  Shift Arithmetic : ArithShift  BitShiftNumber=-8
  Shift Arithmetic1 : ArithShift  BitShiftNumber=-1
  Out1 : Outport
  wires:
  DetectParam1/1 -> Data Type Conversion/1
  Shift Arithmetic/1 -> Bitwise AND/1
  DetectParam2/1 -> Data Type Conversion1/1
  Bitwise AND/1 -> Out1/1
  testEnable/1 -> Data Type Conversion2/1
  Data Type Conversion2/1 -> Bitwise AND/3
  Data Type Conversion/1 -> Shift Arithmetic/1
  Data Type Conversion1/1 -> Shift Arithmetic1/1
  Shift Arithmetic1/1 -> Bitwise AND/2

== system mcb_stm32_param_est_host_read/Algorithm/SerialReceive/Fixed_Point_Target/LatchZero ==
  Status : Inport
  Logical Operator : Logic  AllPortsSameDT=off  OutDataTypeStr=boolean
  Unit Delay : UnitDelay  InitialCondition=1  SampleTime=-1  HasFrameUpgradeWarning=on
  status : Outport
  wires:
  Unit Delay/1 -> Logical Operator/2
  Logical Operator/1 -> Unit Delay/1, status/1
  Status/1 -> Logical Operator/1

== system mcb_stm32_param_est_host_read/Algorithm/SerialReceive/Floating_Point_Target/LatchZero ==
  Status : Inport
  Logical Operator : Logic  AllPortsSameDT=off  OutDataTypeStr=boolean
  Unit Delay : UnitDelay  InitialCondition=1  SampleTime=-1  HasFrameUpgradeWarning=on
  status : Outport
  wires:
  Status/1 -> Logical Operator/1
  Logical Operator/1 -> status/1, Unit Delay/1
  Unit Delay/1 -> Logical Operator/2

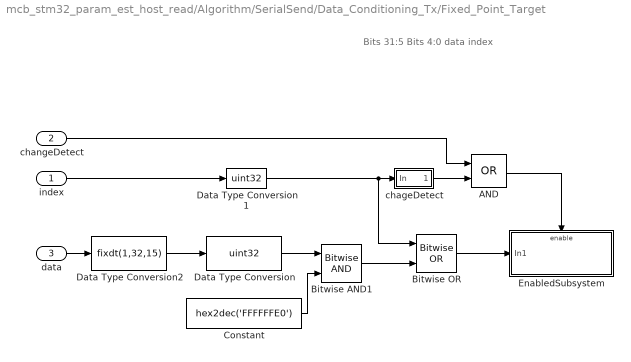
== system mcb_stm32_param_est_host_read/Algorithm/SerialSend/Data_Conditioning_Tx/Fixed_Point_Target ==
  note: Bits 31:5
      | Bits 4:0
      |
      | data
      | index
  index : Inport
  changeDetect : Inport  Port=2
  data : Inport  Port=3
  AND : Logic  Operator=OR  AllPortsSameDT=off  OutDataTypeStr=boolean
  Bitwise AND1 : simulink/Logic and Bit Operations/Bitwise Operator  logicop=AND  UseBitMask=off  NumInputPorts=2  BitMask=hex2dec('fff0')  BitMaskRealWorld=Stored Integer
  Bitwise OR : simulink/Logic and Bit Operations/Bitwise Operator  logicop=OR  UseBitMask=off  NumInputPorts=2  BitMask=bin2dec('11011001')  BitMaskRealWorld=Stored Integer
  Constant : Constant  Value=hex2dec('FFFFFFE0')  OutDataTypeStr=uint32  SampleTime=-1
  Data Type Conversion : DataTypeConversion  OutDataTypeStr=uint32  ConvertRealWorld=Stored Integer (SI)  RndMeth=Simplest  SaturateOnIntegerOverflow=off
  Data Type Conversion1 : DataTypeConversion  OutDataTypeStr=uint32  RndMeth=Simplest  SaturateOnIntegerOverflow=off
  Data Type Conversion2 : DataTypeConversion  OutDataTypeStr=fixdt(1,32,15)  RndMeth=Simplest  SaturateOnIntegerOverflow=off
  EnabledSubsystem : Subsystem  TreatAsAtomicUnit=on
  chageDetect : Subsystem
  wires:
  Constant/1 -> Bitwise AND1/2
  Bitwise AND1/1 -> Bitwise OR/2
  Data Type Conversion/1 -> Bitwise AND1/1
  index/1 -> Data Type Conversion1/1
  Data Type Conversion1/1 -> chageDetect/1(In), Bitwise OR/1
  chageDetect/1(Out) -> AND/2
  changeDetect/1 -> AND/1
  Bitwise OR/1 -> EnabledSubsystem/1(In1)
  AND/1 -> EnabledSubsystem/Enable
  data/1 -> Data Type Conversion2/1
  Data Type Conversion2/1 -> Data Type Conversion/1

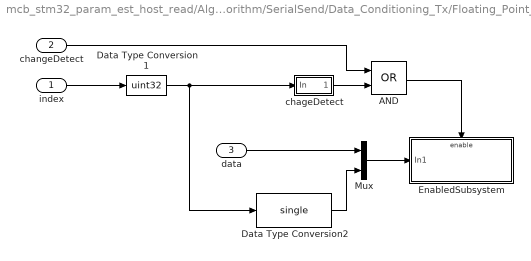
== system mcb_stm32_param_est_host_read/Algorithm/SerialSend/Data_Conditioning_Tx/Floating_Point_Target ==
  index : Inport
  changeDetect : Inport  Port=2
  data : Inport  Port=3
  AND : Logic  Operator=OR  AllPortsSameDT=off  OutDataTypeStr=boolean
  Data Type Conversion1 : DataTypeConversion  OutDataTypeStr=uint32  RndMeth=Simplest  SaturateOnIntegerOverflow=off
  Data Type Conversion2 : DataTypeConversion  OutDataTypeStr=single  RndMeth=Simplest  SaturateOnIntegerOverflow=off
  EnabledSubsystem : Subsystem  TreatAsAtomicUnit=on
  Mux : Mux  Inputs=2
  chageDetect : Subsystem
  wires:
  AND/1 -> EnabledSubsystem/Enable
  changeDetect/1 -> AND/1
  chageDetect/1(Out) -> AND/2
  Data Type Conversion1/1 -> Data Type Conversion2/1, chageDetect/1(In)
  index/1 -> Data Type Conversion1/1
  Data Type Conversion2/1 -> Mux/2
  Mux/1 -> EnabledSubsystem/1(In1)
  data/1 -> Mux/1

== system mcb_stm32_param_est_host_read/Algorithm/SignalConditioning/LatchIdx/Enabled Subsystem ==
  status : Inport
  Enable : EnablePort
  Idx : Outport
  wires:
  status/1 -> Idx/1

== system mcb_stm32_param_est_host_read/Algorithm/SignalConditioning/Subsystem1/Switch Case Action Subsystem1 ==
  In1 : Inport
  Action Port : ActionPort  InitializeStates=reset  ActionPortLabel=case [ 8 ]:
  Out1 : Outport
  wires:
  In1/1 -> Out1/1

== system mcb_stm32_param_est_host_read/Algorithm/SignalConditioning/Subsystem1/Switch Case Action Subsystem10 ==
  In1 : Inport
  Action Port : ActionPort  ActionPortLabel=case [ 7 ]:
  To Workspace : ToWorkspace  VariableName=B  SampleTime=-1
      settings: MaxDataPoints=1  Save2DSignal=2-D array (concatenate along first dimension)
  wires:
  In1/1 -> To Workspace/1

== system mcb_stm32_param_est_host_read/Algorithm/SignalConditioning/Subsystem1/Switch Case Action Subsystem11 ==
  Action Port : ActionPort  ActionPortLabel=default:

== system mcb_stm32_param_est_host_read/Algorithm/SignalConditioning/Subsystem1/Switch Case Action Subsystem2 ==
  In1 : Inport
  Action Port : ActionPort  ActionPortLabel=case [ 3 ]:
  To Workspace : ToWorkspace  VariableName=Ld  SampleTime=-1
      settings: MaxDataPoints=1  Save2DSignal=2-D array (concatenate along first dimension)
  wires:
  In1/1 -> To Workspace/1

== system mcb_stm32_param_est_host_read/Algorithm/SignalConditioning/Subsystem1/Switch Case Action Subsystem3 ==
  In1 : Inport
  Action Port : ActionPort  ActionPortLabel=case [ 4 ]:
  To Workspace : ToWorkspace  VariableName=Lq  SampleTime=-1
      settings: MaxDataPoints=1  Save2DSignal=2-D array (concatenate along first dimension)
  wires:
  In1/1 -> To Workspace/1

== system mcb_stm32_param_est_host_read/Algorithm/SignalConditioning/Subsystem1/Switch Case Action Subsystem4 ==
  In1 : Inport
  Action Port : ActionPort  ActionPortLabel=case [ 1 ]:
  Gain : Gain  Gain=1e4  RndMeth=Simplest  OutDataTypeStr=Inherit: Same as input
  To Workspace : ToWorkspace  VariableName=Ib_avg_cal  SampleTime=-1
      settings: MaxDataPoints=1  Save2DSignal=2-D array (concatenate along first dimension)
  wires:
  In1/1 -> Gain/1
  Gain/1 -> To Workspace/1

== system mcb_stm32_param_est_host_read/Algorithm/SignalConditioning/Subsystem1/Switch Case Action Subsystem5 ==
  In1 : Inport
  Action Port : ActionPort  ActionPortLabel=case [ 0 ]:
  Gain : Gain  Gain=1e4  RndMeth=Simplest  OutDataTypeStr=Inherit: Same as input
  To Workspace : ToWorkspace  VariableName=Ia_avg_cal  SampleTime=-1
      settings: MaxDataPoints=1  Save2DSignal=2-D array (concatenate along first dimension)
  wires:
  In1/1 -> Gain/1
  Gain/1 -> To Workspace/1

== system mcb_stm32_param_est_host_read/Algorithm/SignalConditioning/Subsystem1/Switch Case Action Subsystem6 ==
  In1 : Inport
  Action Port : ActionPort  ActionPortLabel=case [ 9 ]:
  Terminator : Terminator
  wires:
  In1/1 -> Terminator/1

== system mcb_stm32_param_est_host_read/Algorithm/SignalConditioning/Subsystem1/Switch Case Action Subsystem7 ==
  In1 : Inport
  Action Port : ActionPort  ActionPortLabel=case [ 2 ]:
  To Workspace : ToWorkspace  VariableName=Rs  SampleTime=-1
      settings: MaxDataPoints=1  Save2DSignal=2-D array (concatenate along first dimension)
  wires:
  In1/1 -> To Workspace/1

== system mcb_stm32_param_est_host_read/Algorithm/SignalConditioning/Subsystem1/Switch Case Action Subsystem8 ==
  In1 : Inport
  Action Port : ActionPort  ActionPortLabel=case [ 5 ]:
  To Workspace : ToWorkspace  VariableName=Ke  SampleTime=-1
      settings: MaxDataPoints=1  Save2DSignal=2-D array (concatenate along first dimension)
  wires:
  In1/1 -> To Workspace/1

== system mcb_stm32_param_est_host_read/Algorithm/SignalConditioning/Subsystem1/Switch Case Action Subsystem9 ==
  In1 : Inport
  Action Port : ActionPort  ActionPortLabel=case [ 6 ]:
  To Workspace : ToWorkspace  VariableName=J  SampleTime=-1
      settings: MaxDataPoints=1  Save2DSignal=2-D array (concatenate along first dimension)
  wires:
  In1/1 -> To Workspace/1

== system mcb_stm32_param_est_host_read/Algorithm/SerialSend/Data_Conditioning_Tx/Fixed_Point_Target/EnabledSubsystem ==
  In1 : Inport
  Enable : EnablePort
  Host Serial Transmit : instrumentseriallib/Serial Send  PortSel=COM8  Port=COM8  ComPort=COM8  Header=[]  Terminator=<none>  CustomTerminator=[]  EnableBlockingMode=off  SimulateUsing=Interpreted execution  BlockInModel=on  aMode=5
  wires:
  In1/1 -> Host Serial Transmit/1

== system mcb_stm32_param_est_host_read/Algorithm/SerialSend/Data_Conditioning_Tx/Fixed_Point_Target/chageDetect ==
  In : Inport
  Relational Operator4 : RelationalOperator  Operator=~=  OutDataTypeStr=boolean  InputSameDT=off
  Unit Delay4 : UnitDelay  SampleTime=-1  HasFrameUpgradeWarning=on
  Out : Outport
  wires:
  In/1 -> Unit Delay4/1, Relational Operator4/1
  Unit Delay4/1 -> Relational Operator4/2
  Relational Operator4/1 -> Out/1

== system mcb_stm32_param_est_host_read/Algorithm/SerialSend/Data_Conditioning_Tx/Floating_Point_Target/EnabledSubsystem ==
  In1 : Inport
  Enable : EnablePort
  Host Serial Transmit : instrumentseriallib/Serial Send  PortSel=COM8  Port=COM8  ComPort=COM8  Header=''  Terminator=<none>  CustomTerminator='EEDD'  EnableBlockingMode=off  SimulateUsing=Interpreted execution  BlockInModel=on  aMode=5
  wires:
  In1/1 -> Host Serial Transmit/1

== system mcb_stm32_param_est_host_read/Algorithm/SerialSend/Data_Conditioning_Tx/Floating_Point_Target/chageDetect ==
  In : Inport
  Relational Operator4 : RelationalOperator  Operator=~=  OutDataTypeStr=boolean  InputSameDT=off
  Unit Delay4 : UnitDelay  SampleTime=-1  HasFrameUpgradeWarning=on
  Out : Outport
  wires:
  Relational Operator4/1 -> Out/1
  Unit Delay4/1 -> Relational Operator4/2
  In/1 -> Relational Operator4/1, Unit Delay4/1

== matlab function mcb_stm32_param_est_host_read/Algorithm/SignalConditioning/Data_Conditioning2 ==
  data: rawInput input; selSignal output
function selSignal = fcn(rawInput)

selSignal = rawInput(:, 2);

end

== matlab function mcb_stm32_param_est_host_read/Algorithm/SignalConditioning/ErrorConditions ==
  data: status input; idx input; errorID input
function fcn(status, idx, errorID)

%   Copyright 2019 The MathWorks, Inc.

coder.extrinsic('message', 'msgbox', 'set_param', 'error', 'isempty');

persistent prev_idx
if isempty(prev_idx)
	prev_idx = single(20);
end

% host model will be stopped under the following conditions
% 
% 1. if estiamtion algorithm sends an error signal
% 2. if serial communication status fails 
% 3. if all tests are done and all parameters are sent from the target
% model
if errorID || ~status || (idx == 9 && prev_idx == 7)
    
    set_param(bdroot, 'SimulationCommand','stop');
    if errorID == 1
        (error(message('mcb:blocks:OverCurrentDetected')));
    elseif errorID == 2
        (error(message('mcb:blocks:UnderVoltageDetected')));
    end
    if ~status
        (error(message('mcb:blocks:SerialComFailure')));
    end
end

if ~isequal(idx, prev_idx)
	prev_idx = idx;
end

== matlab function mcb_stm32_param_est_host_read/Algorithm/SignalConditioning/Data_Conditioning1 ==
  data: unused input; estParamIdx output; estParam output; rawInput input
function [ estParamIdx, estParam] = estParam(~, rawInput)

% Odd - EstParamIdx;  Even - EstParam
persistent estParamIdxOut;
if isempty(estParamIdxOut)
    estParamIdxOut = single(20);
end
persistent estParamOut;
if isempty(estParamOut)
    estParamOut = single(0);
end
persistent flag;
if isempty(flag)
    flag = single(0);
end
if estParamIdxOut~= rawInput(1,1) || flag
    if length(unique(rawInput(1:2:19,1))) == 1 && length(unique(rawInput(2:2:20,1))) == 1
        estParamIdxOut = rawInput(1,1);
        estParamOut = rawInput(2,1);
        flag = single(0);
    elseif length(unique(rawInput(301:2:319,1))) == 1 && length(unique(rawInput(302:2:320,1))) == 1
        estParamIdxOut = rawInput(301,1);
        estParamOut = rawInput(302,1);
        flag = single(0);
    elseif length(unique(rawInput(581:2:599,1))) == 1 && length(unique(rawInput(582:2:600,1))) == 1
        estParamIdxOut = rawInput(581,1);
        estParamOut = rawInput(582,1);
        flag = single(0);
    else
        flag = single(1);
    end
end

estParamIdx = estParamIdxOut;
estParam = estParamOut;
end

== matlab function mcb_stm32_param_est_host_read/Algorithm/SerialReceive/Floating_Point_Target/checkStatus ==
  data: Data input; ErrorCode input; Status output
function Status = checkStatus(Data, ErrorCode)

% Status = ~(any(Data(:) == ErrorCode));
% if ~Status
%     disp('error');
% end
errIdx = find(Data(:) == ErrorCode);
Status = ~(numel(errIdx) > 10);
% persistent errNumStatus;
% if isempty(errNumStatus)
%     errNumStatus = 0;
% end
% 
% errStatus = ~(any(Data(:) == ErrorCode));
% Status = true;
% if errStatus
%     errNumStatus = errNumStatus + 1;
% else
%     if errNumStatus > 3
%         Status = false;
%     else
%         errNumStatus = 0;
%         Status = true;
%     end
%     
% end

end

== matlab function mcb_stm32_param_est_host_read/Algorithm/SerialReceive/Fixed_Point_Target/checkStatus ==
  data: Data input; ErrorCode input; Status output
function Status = checkStatus(Data, ErrorCode)

Status = ~(any(Data(:) == ErrorCode));

end
